simulink model "no2_proportional_controller_steady_state_error"  (R2025a)
settings: Solver=VariableStepAuto  StartTime=0.0  StopTime=Inf  RelTol=1e-3
libraries: simulink x1
settings Model: Creator=ayeo  LastModifiedBy=ayeo

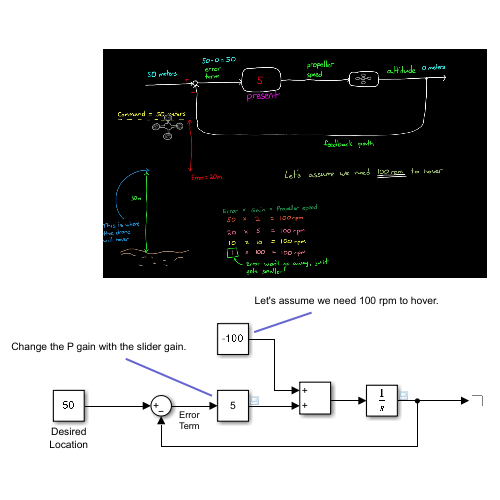
[thumbnail: Simulink's stored preview of the top-level diagram]
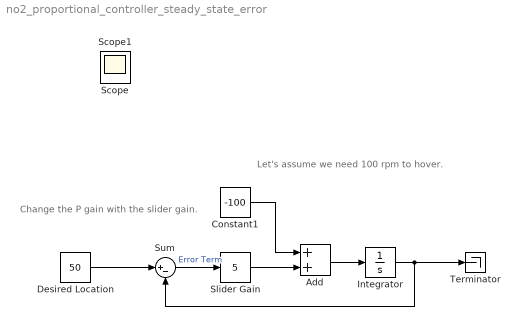
== system no2_proportional_controller_steady_state_error ==
  note: Let's assume we need 100 rpm to hover.
  note: Change the P gain with the slider gain.
  Add : Sum
  Constant1 : Constant  Value=-100
  Desired Location : Constant  Value=50
  Integrator : Integrator
  Slider Gain : simulink/Math Operations/Slider Gain  gain=5  low=2  high=100
  Sum : Sum  Inputs=|+-
  Terminator : Terminator
  Scope : Scope
      settings: ActiveDisplayYMinimum=-6.0531292843981808  ActiveDisplayYMaximum=54.478163559583656
  Scope1 : Scope
      settings: ActiveDisplayYMinimum=99.999999999999986  ActiveDisplayYMaximum=100.00000000000001
  wires:
  Desired Location/1 -> Sum/1
  Sum/1 -> Slider Gain/1  "Error Term"
  Slider Gain/1 -> Add/2
  Integrator/1 -> Sum/2, Terminator/1
  Add/1 -> Integrator/1
  Constant1/1 -> Add/1
